simulink model "lab1ex8"  (Simulink 6.0)
settings: Solver=ode45  StartTime=0.0  StopTime=10.0  RelTol=1e-3
undefined symbols (not defined in the file): k, z
settings Model: LastModifiedBy=student

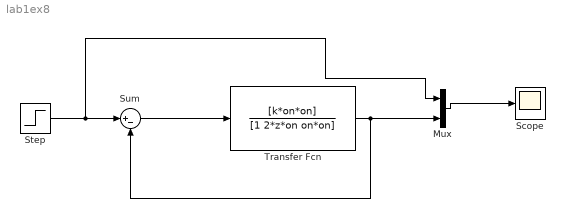
== system lab1ex8 ==
  Mux : Mux  Inputs=2
  Scope : Scope
  Step : Step  SampleTime=0
  Sum : Sum  Inputs=|+-
  Transfer Fcn : TransferFcn  Numerator=[k*on*on]  Denominator=[1 2*z*on on*on]
  wires:
  Transfer Fcn/1 -> Mux/2, Sum/2
  Mux/1 -> Scope/1
  Sum/1 -> Transfer Fcn/1
  Step/1 -> Sum/1, Mux/1
